simulink model "estabilidade"  (Simulink 7.1)
settings: Solver=ode45  StartTime=0.0  StopTime=70  RelTol=1e-3
settings Model: Creator=CARLOS BRUNO  LastModifiedBy=CARLOS BRUNO

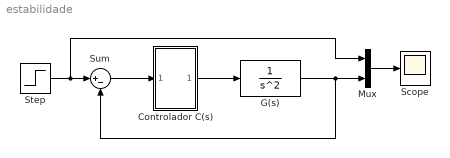
== system estabilidade ==
  Controlador C(s) : Subsystem  mask{K=0.0324, a=0.588}
      mask prompts: K "variavel K"; a "variavel a"
  G(s) : TransferFcn  Denominator=[1 0 0]
  Mux : Mux  Inputs=2
  Scope : Scope
  Step : Step  Time=0  SampleTime=0
  Sum : Sum  Inputs=|+-  OutDataType=sfix(16)  OutScaling=2^0
  wires:
  G(s)/1 -> Sum/2, Mux/2
  Sum/1 -> Controlador C(s)/1(In1)
  Controlador C(s)/1(Out1) -> G(s)/1
  Step/1 -> Sum/1, Mux/1
  Mux/1 -> Scope/1

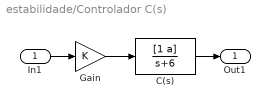
== system estabilidade/Controlador C(s) ==
  In1 : Inport
  C(s) : TransferFcn  Numerator=[1 a]  Denominator=[1 6]
  Gain : Gain  Gain=K  ParameterDataType=sfix(16)  ParameterScaling=2^0  OutDataType=sfix(16)  OutScaling=2^0
  Out1 : Outport
  wires:
  Gain/1 -> C(s)/1
  C(s)/1 -> Out1/1
  In1/1 -> Gain/1
